simulink model "LQR_ydx_control"  (R2022b)
settings: Solver=VariableStepAuto  StartTime=0.0  StopTime=150  RelTol=1e-3
values from neighbouring files (symbols this model uses):
  cx = 0:0.1:120    [lqrydx_ref_01.m]
libraries: Solver_SF x2, simulink x2
settings Model: Creator=admin  LastModifiedBy=admin

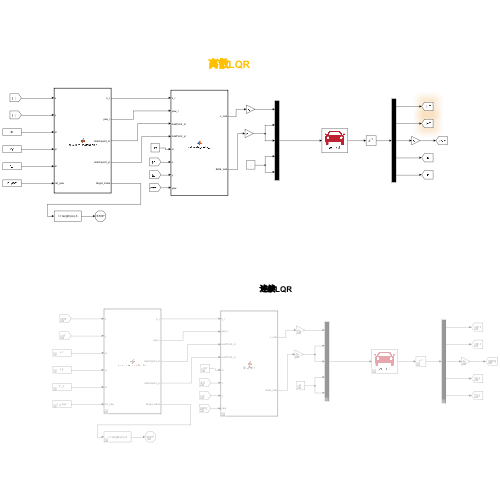
[thumbnail: Simulink's stored preview of the top-level diagram]
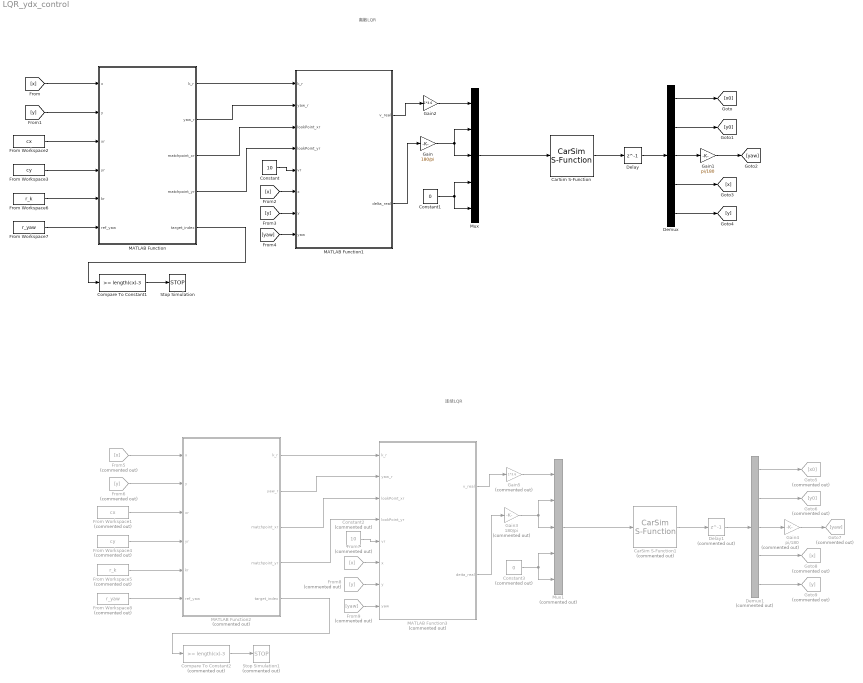
== system LQR_ydx_control ==
  note: 连续LQR
  note: 离散LQR
  CarSim S-Function : Solver_SF/CarSim S-Function  Priority=1  SIMFILE=simfile.sim  Run_RTs=off  vs_state_ind=Run  StopMode_ind=Vehicle Model
  CarSim S-Function1 : Solver_SF/CarSim S-Function  Priority=1  Commented=on  SIMFILE=simfile.sim  Run_RTs=off  vs_state_ind=Run  StopMode_ind=Vehicle Model
  Compare To Constant1 : simulink/Logic and Bit Operations/Compare To Constant  relop=>=  const=length(cx)-3  OutDataTypeStr=boolean
  Compare To Constant2 : simulink/Logic and Bit Operations/Compare To Constant  Commented=on  relop=>=  const=length(cx)-3  OutDataTypeStr=boolean
  Constant : Constant  Value=10
  Constant1 : Constant  Value=0
  Constant2 : Constant  Commented=on  Value=10
  Constant3 : Constant  Commented=on  Value=0
  Delay : Delay  DelayLength=1
  Delay1 : Delay  Commented=on  DelayLength=1
  Demux : Demux  Outputs=5
  Demux1 : Demux  Commented=on  Outputs=5
  From Workspace1 : FromWorkspace  Commented=on  VariableName=cx
  From Workspace2 : FromWorkspace  VariableName=cx
  From Workspace3 : FromWorkspace  VariableName=cy
  From Workspace4 : FromWorkspace  Commented=on  VariableName=cy
  From Workspace5 : FromWorkspace  Commented=on  VariableName=r_k
  From Workspace6 : FromWorkspace  VariableName=r_k
  From Workspace7 : FromWorkspace  VariableName=r_yaw
  From Workspace8 : FromWorkspace  Commented=on  VariableName=r_yaw
  From5 : From  Commented=on  GotoTag=x
  From6 : From  Commented=on  GotoTag=y
  From7 : From  Commented=on  GotoTag=x
  From8 : From  Commented=on  GotoTag=y
  From9 : From  Commented=on  GotoTag=yaw
  Gain : Gain  Gain=180/pi
  Gain1 : Gain  Gain=pi/180
  Gain2 : Gain  Gain=1*3.6
  Gain3 : Gain  Commented=on  Gain=180/pi
  Gain4 : Gain  Commented=on  Gain=pi/180
  Gain5 : Gain  Commented=on  Gain=1*3.6
  Goto5 : Goto  Commented=on  GotoTag=x0
  Goto6 : Goto  Commented=on  GotoTag=y0
  Goto7 : Goto  Commented=on  GotoTag=yaw
  Goto8 : Goto  Commented=on  GotoTag=x
  Goto9 : Goto  Commented=on  GotoTag=y
  MATLAB Function : MATLAB Function  TreatAsAtomicUnit=on
  MATLAB Function1 : MATLAB Function  TreatAsAtomicUnit=on
  MATLAB Function2 : MATLAB Function  Commented=on  TreatAsAtomicUnit=on
  MATLAB Function3 : MATLAB Function  Commented=on  TreatAsAtomicUnit=on
  Mux : Mux  Inputs=5
  Mux1 : Mux  Commented=on  Inputs=5
  Stop Simulation : Stop
  Stop Simulation1 : Stop  Commented=on
  wires:
  Gain2/1 -> Mux/1
  Gain/1 -> Mux/3, Mux/2
  Constant1/1 -> Mux/4, Mux/5
  Demux/1 -> [x0]
  Demux/2 -> [y0]
  Demux/3 -> Gain1/1
  Gain1/1 -> [yaw]
  Demux/4 -> [x]
  Demux/5 -> [y]
  [x] -> MATLAB Function/1(x)
  [y] -> MATLAB Function/2(y)
  From Workspace2/1 -> MATLAB Function/3(xr)
  From Workspace3/1 -> MATLAB Function/4(yr)
  From Workspace6/1 -> MATLAB Function/5(kr)
  From Workspace7/1 -> MATLAB Function/6(ref_yaw)
  Mux/1 -> CarSim S-Function/1
  CarSim S-Function/1 -> Delay/1
  Delay/1 -> Demux/1
  MATLAB Function/5(target_index) -> Compare To Constant1/1
  Compare To Constant1/1 -> Stop Simulation/1
  MATLAB Function/1(k_r) -> MATLAB Function1/1(k_r)
  MATLAB Function/2(yaw_r) -> MATLAB Function1/2(yaw_r)
  MATLAB Function/3(matchpoint_xr) -> MATLAB Function1/3(lookPoint_xr)
  MATLAB Function/4(matchpoint_yr) -> MATLAB Function1/4(lookPoint_yr)
  [x] -> MATLAB Function1/6(x)
  [y] -> MATLAB Function1/7(y)
  [yaw] -> MATLAB Function1/8(yaw)
  Constant/1 -> MATLAB Function1/5(vr)
  MATLAB Function1/1(v_real) -> Gain2/1
  MATLAB Function1/2(delta_real) -> Gain/1
  From Workspace1/1 -> MATLAB Function2/3(xr)
  From Workspace4/1 -> MATLAB Function2/4(yr)
  MATLAB Function3/2(deita_real) -> Gain3/1
  Mux1/1 -> CarSim S-Function1/1
  Delay1/1 -> Demux1/1
  Constant2/1 -> MATLAB Function3/5(vr)
  MATLAB Function2/3(matchpoint_xr) -> MATLAB Function3/3(lookPoint_xr)
  From9/1 -> MATLAB Function3/8(yaw)
  MATLAB Function2/2(yaw_r) -> MATLAB Function3/2(yaw_r)
  Gain3/1 -> Mux1/3, Mux1/2
  MATLAB Function2/4(matchpoint_yr) -> MATLAB Function3/4(lookPoint_yr)
  From5/1 -> MATLAB Function2/1(x)
  From7/1 -> MATLAB Function3/6(x)
  MATLAB Function3/1(v_real) -> Gain5/1
  From Workspace5/1 -> MATLAB Function2/5(kr)
  MATLAB Function2/1(k_r) -> MATLAB Function3/1(k_r)
  Demux1/1 -> Goto5/1
  Demux1/4 -> Goto8/1
  Demux1/3 -> Gain4/1
  Demux1/5 -> Goto9/1
  CarSim S-Function1/1 -> Delay1/1
  From Workspace8/1 -> MATLAB Function2/6(ref_yaw)
  Gain4/1 -> Goto7/1
  From6/1 -> MATLAB Function2/2(y)
  Constant3/1 -> Mux1/4, Mux1/5
  Gain5/1 -> Mux1/1
  MATLAB Function2/5(target_index) -> Compare To Constant2/1
  From8/1 -> MATLAB Function3/7(y)
  Demux1/2 -> Goto6/1
  Compare To Constant2/1 -> Stop Simulation1/1

== matlab function LQR_ydx_control/MATLAB Function1 ==
  data: k_r input; v_real output; yaw_r input; lookPoint_xr input; lookPoint_yr input; vr input; x input; y input; yaw input; delta_real output
function [v_real, delta_real] = calculate_delta_f(k_r,yaw_r,lookPoint_xr, lookPoint_yr,vr,x,y,yaw)
    L=2.6;                           %车长
    r_Delta = atan(L*k_r);           %参考的前轮转角，有固定公式
    
    x_error  = x - lookPoint_xr;     %x方向误差
    y_error = y - lookPoint_yr;      %y方向误差
    yaw_error =  yaw - yaw_r;        %横摆角误差
    e_X=[x_error;y_error;yaw_error]; %状态方程中的状态，即 x误差,y误差,横摆角误差
    
    %% 离散状态空间方程：Xk+1=AXk+Buk 对应的矩阵
    dt=0.05;                         %仿真步长
    A = [1,  0,  -vr*dt*sin(yaw_r);
         0,  1,  vr * dt * cos(yaw_r);
         0,  0,  1];
    B = [dt * cos(yaw_r),    0;
         dt * sin(yaw_r),    0;
         dt * tan(yaw_r)/L,  vr*dt/(L * cos(r_Delta)^2)];
    %% 目标函数对应的Q,R矩阵设置
    Q=[200,  0,  0;                  %权重矩阵Q
         0,  200,  0;
         0,  0,  80];
    
    R=[7,  0;                        %权重矩阵R
         0,  20];
    
    %% 求解P矩阵，稳住，按给定步骤求解即可
    % 终止条件定义
    iter_max = 500;                  %最大迭代次数
    epsilon = 0.01;                  %允许误差
    
    P_old = Q;
    for i = 1:iter_max
        P_new = A' * P_old * A - (A' * P_old * B)/(R + B' * P_old * B) *( B' * P_old * A) +Q;
        if abs(P_new - P_old) <= epsilon
            break
        else
            P_old = P_new; 
        end
    end
    
    P = P_new;                       %最终P矩阵
    %% 求得P矩阵后，根据公式，得到状态反馈增益K,并得到控制律
    K = (B' * P * B + R) \ (B' * P * A);  
    u = -K * e_X;                    %控制率，u=-kx，2行1列
    %% 最终转换
    v_delta = u(1);      
    Delta_delta = u(2);
    
    v_real=vr+v_delta;                  %最终控制量速度：V
    delta_real=r_Delta+Delta_delta;     %最终控制量前轮转角：deita
end

== matlab function LQR_ydx_control/MATLAB Function ==
  data: x input; k_r output; y input; xr input; yr input; kr input; ref_yaw input; yaw_r output; matchpoint_xr output; matchpoint_yr output; target_index output
function [k_r, yaw_r, matchpoint_xr, matchpoint_yr, target_index] = calculate_matchpoint(x,y,xr,yr,kr,ref_yaw)
    total_point = length(xr);
    min_distance = (xr(1) - x)^2 + (yr(1) - y)^2;
    min_index = 0;
    for i = 1:total_point
        distance = (xr(i) - x)^2 + (yr(i) - y)^2;
        if distance < min_distance
           min_distance = distance;
           min_index = i;
        end
    end

    if min_index <=1
        min_index = 1;
    end

    target_index = min_index;
    matchpoint_xr = xr(target_index);
    matchpoint_yr = yr(target_index);
    k_r = kr(target_index);
    yaw_r = ref_yaw(target_index);
end

== matlab function LQR_ydx_control/MATLAB Function2 ==
  data: x input; k_r output; y input; xr input; yr input; kr input; ref_yaw input; yaw_r output; matchpoint_xr output; matchpoint_yr output; target_index output
function [k_r, yaw_r, matchpoint_xr, matchpoint_yr, target_index] = calculate_matchpoint(x,y,xr,yr,kr,ref_yaw)
    total_point = length(xr);
    min_distance = (xr(1) - x)^2 + (yr(1) - y)^2;
    min_index = 0;
    for i = 1:total_point
        distance = (xr(i) - x)^2 + (yr(i) - y)^2;
        if distance < min_distance
           min_distance = distance;
           min_index = i;
        end
    end

    if min_index <=1
        min_index = 1;
    end

    target_index = min_index;
    matchpoint_xr = xr(target_index);
    matchpoint_yr = yr(target_index);
    k_r = kr(target_index);
    yaw_r = ref_yaw(target_index);
end

== matlab function LQR_ydx_control/MATLAB Function3 ==
  data: k_r input; v_real output; yaw_r input; lookPoint_xr input; lookPoint_yr input; vr input; x input; y input; yaw input; deita_real output
function [v_real,deita_real] = findPoint(k_r,yaw_r,lookPoint_xr, lookPoint_yr,vr,x,y,yaw)

L=2.6;                              %车长
r_Delta = atan(L*k_r);              %参考的前轮转角

x_error  = x - lookPoint_xr;        %x方向误差
y_error = y - lookPoint_yr;         %y方向误差
yaw_error =  yaw - yaw_r;           %横摆角误差
e_X=[x_error;y_error;yaw_error];    %状态方程中的状态

% X=AX+Bu 由状态方程系数矩阵
A = [0,  0,  -vr*sin(yaw_r);
     0,  0,  vr* cos(yaw_r);
     0,  0,  0];
B = [ cos(yaw_r),    0;
      sin(yaw_r),    0;
     tan(yaw_r)/L,  vr/(L * cos(r_Delta)^2)];

Q=[200,  0,  0;                     %权重矩阵Q
     0,  200,  0;
     0,  0,  80];
R=[7,  0;                           %权重矩阵R
     0,  20];

coder.extrinsic('lqr');             %此代码使在MATLAB function模块中可以使用求解工具lqr()
K=[ 0,    0,   0;
    0,    0,   0];
K = lqr(A,B,Q,R);                   %使用MATLAB工具求K

u = -K * e_X;                       %由反馈K得出最终控制量：u=-Kx

%控制律最终转换
v_delta = u(1);      
Delta_delta = u(2);
v_real=vr+v_delta;                  %最终控制量速度：V
deita_real=r_Delta+Delta_delta;     %最终控制量前轮转角：deita
end
